simulink model "PI_OL_vs_PI_CC_v2023b"  (R2023b)
settings: Solver=FixedStepDiscrete  StartTime=0.0  StopTime=30  FixedStep=Ts_Power  MaxStep=1e-4  RelTol=1e-3
InitFcn:
  | run PI_VC_vs_PI_CC_ini;
values from neighbouring files (symbols this model uses):
  C = 4e-6    (= 4e-06)    [PI_OL_vs_PI_CC_ini.m]    (also in PI_VC_vs_UPI_CC_ini.m)
  C_2 = 4e-6    (= 4e-06)    [PI_OL_vs_PI_CC_ini.m]    (also in PI_VC_vs_UPI_CC_ini.m)
  K_i_pll = 1.8/0.00251    (= 717.131474104)    [PI_OL_vs_PI_CC_ini.m]    (also in PI_VC_vs_UPI_CC_ini.m)
  K_p_pll = 1.8    [PI_OL_vs_PI_CC_ini.m]    (also in PI_VC_vs_UPI_CC_ini.m)
  L_line_12_13 = X_line_12_13/(2*pi*50)    (= 0.000798957814321)    [PI_OL_vs_PI_CC_ini.m]    (also in PI_VC_vs_UPI_CC_ini.m)
  L_line_13_14 = X_line_13_14/(2*pi*50)    (= 0.000200535228296)    [PI_OL_vs_PI_CC_ini.m]    (also in PI_VC_vs_UPI_CC_ini.m)
  L_s = 1.25e-3    (= 0.00125)    [PI_OL_vs_PI_CC_ini.m]    (also in PI_VC_vs_UPI_CC_ini.m)
  L_s2 = 1.25e-3    (= 0.00125)    [PI_OL_vs_PI_CC_ini.m]    (also in PI_VC_vs_UPI_CC_ini.m)
  L_t = 1.25e-3    (= 0.00125)    [PI_OL_vs_PI_CC_ini.m]    (also in PI_VC_vs_UPI_CC_ini.m)
  L_t2 = 1.25e-3    (= 0.00125)    [PI_OL_vs_PI_CC_ini.m]    (also in PI_VC_vs_UPI_CC_ini.m)
  params_cc = [R_t2;L_t2;R_s2;L_s2;K_pi;Ki_i]    [PI_OL_vs_PI_CC_ini.m]    (also in PI_VC_vs_UPI_CC_ini.m)
  params_pi_cc = [S_b,U_b,K_p,T_p,K_q,T_q,X,R]    [PI_OL_vs_PI_CC_ini.m]    (also in PI_VC_vs_UPI_CC_ini.m)
  params_pi_vc = [S_b,U_b,K_p,T_p,K_q,T_q,Xv,Rv]    [PI_OL_vs_PI_CC_ini.m]    (also in PI_VC_vs_UPI_CC_ini.m)
  R_d = 10    [PI_OL_vs_PI_CC_ini.m]    (also in PI_VC_vs_UPI_CC_ini.m)
  R_d2 = 10    [PI_OL_vs_PI_CC_ini.m]    (also in PI_VC_vs_UPI_CC_ini.m)
  R_line_12_13 = (0.06)*Length    (= 0.24)    [PI_OL_vs_PI_CC_ini.m]    (also in PI_VC_vs_UPI_CC_ini.m)
  R_line_13_14 = (0.025)*Length    (= 0.1)    [PI_OL_vs_PI_CC_ini.m]    (also in PI_VC_vs_UPI_CC_ini.m)
  R_s = L_s*omega/10    (= 0.0392699081699)    [PI_OL_vs_PI_CC_ini.m]    (also in PI_VC_vs_UPI_CC_ini.m)
  R_s2 = L_s*omega/10    (= 0.0392699081699)    [PI_OL_vs_PI_CC_ini.m]    (also in PI_VC_vs_UPI_CC_ini.m)
  R_t = L_t*omega/10    (= 0.0392699081699)    [PI_OL_vs_PI_CC_ini.m]    (also in PI_VC_vs_UPI_CC_ini.m)
  R_t2 = L_t*omega/10    (= 0.0392699081699)    [PI_OL_vs_PI_CC_ini.m]    (also in PI_VC_vs_UPI_CC_ini.m)
  S_b = 20e3    (= 20000)    [PI_OL_vs_PI_CC_ini.m]    (also in PI_VC_vs_UPI_CC_ini.m)
  Ts_Control = 50e-6    (= 5e-05)    [PI_OL_vs_PI_CC_ini.m]    (also in PI_VC_vs_UPI_CC_ini.m)
  Ts_Power = 50e-6    (= 5e-05)    [PI_OL_vs_PI_CC_ini.m]    (also in PI_VC_vs_UPI_CC_ini.m)
  v_dc = 800    [PI_OL_vs_PI_CC_ini.m]    (also in PI_VC_vs_UPI_CC_ini.m)
undefined symbols (not defined in the file or in its folder): DiscIntNeverNeededParam
libraries: spsThreePhaseSeriesRLCBranchLib x10, spsThreePhaseVIMeasurementLib x6, spsFirstOrderFilterLib x4, eeGeneralControl x2, spsPower3phInstantaneousLib x2, spsDCVoltageSourceLib x2, spsUniversalBridgeLib x2, spsVoltageMeasurementLib x2, spsThreePhaseBreakerLib x2, spsRMSLib x1, simulink x1, spsGroundLib x1
settings Model: Creator=Manuel  LastModifiedBy=iberi
settings SolverCC: AlgebraicLoopSolver=TrustRegion
settings DataIOCC: ReturnWorkspaceOutputs=off
settings DebuggingCC: UnconnectedInputMsg=warning  UnconnectedOutputMsg=warning  UnconnectedLineMsg=warning  ArithmeticOperatorsInVariantConditions=warning
settings ModelReferenceCC: EnableRefExpFcnMdlSchedulingChecks=on
settings SFSimCC: SimUseLocalCustomCode=off  CustomCodeUndefinedFunction=UseInterfaceOnly
settings RTWCC: RTWUseLocalCustomCode=off  DLArmComputeVersion=19.05

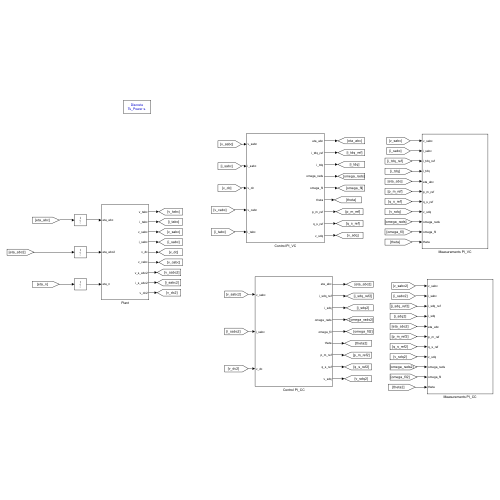
[thumbnail: Simulink's stored preview of the top-level diagram]
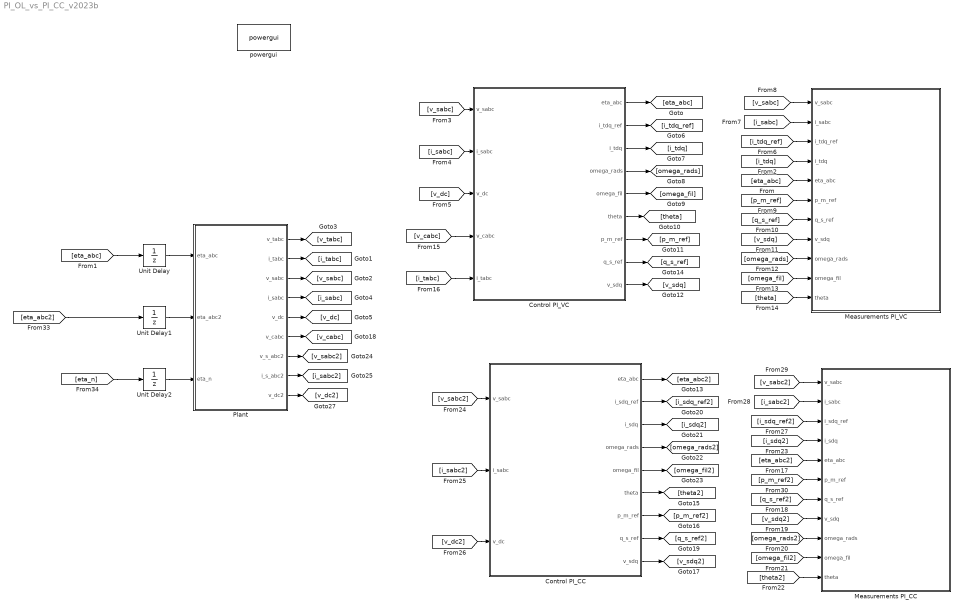
== system PI_OL_vs_PI_CC_v2023b ==
  Control PI_CC : Subsystem
  Control PI_VC : Subsystem
  Measurements PI_CC : Subsystem
  Measurements PI_VC : Subsystem
  Plant : Subsystem
  Unit Delay : UnitDelay  SampleTime=-1  HasFrameUpgradeWarning=on
  Unit Delay1 : UnitDelay  SampleTime=-1  HasFrameUpgradeWarning=on
  Unit Delay2 : UnitDelay  SampleTime=-1  HasFrameUpgradeWarning=on
  powergui : spspowerguiLib/powergui  Priority=1  SimulationMode=Discrete  SampleTime=Ts_Power  frequency=60  Iterations=50  frequencyindice=0  Pbase=100e6  ErrMax=1e-4  UnitsV=kV  UnitsW=MW  buscounter=0  FunctionMessages=off  echomessages=off  EnableUseOfTLC=off  CurrentSourceSwitches=off  DisableSnubberDevices=off  DisableRonSwitches=off  DisableVfSwitches=off  DisplayEquations=off  AutomaticDiscreteSolvers=off  SolverType=Tustin/Backward Euler (TBE)  Interpol=off  ExternalGateDelay=off  methode=off  Ts=100  x0status=blocks  SPID=on  SwTol=0  HookPort=off  NonlinearTolerance=1e-4  nMaxIteration=100  ContinueOnMaxIteration=off  RestoreLinks=warning  ResistiveCurrentMeasurement=off  Frange=[0:2:500]  Ylog=off  Xlog=on  ShowGrid=off  save=off  variable=ZData  structure=v_sabc  ZoomFFT=off  StartTime=4  cycles=5  DisplayStyle=2  fundamental=50  FreqAxis=off  MaxFrequency=10000  frequencyindicesteady=1  RmsSteady=1  display=off
  wires:
  Plant/5(v_dc) -> [v_dc]
  [eta_abc] -> Unit Delay/1
  Plant/1(v_tabc) -> [v_tabc]
  Plant/2(i_tabc) -> [i_tabc]
  Plant/4(i_sabc) -> [i_sabc]
  Plant/3(v_sabc) -> [v_sabc]
  Plant/6(v_cabc) -> [v_cabc]
  [v_sabc] -> Control PI_VC/1(v_sabc)
  [i_sabc] -> Control PI_VC/2(i_sabc)
  [v_dc] -> Control PI_VC/3(v_dc)
  Control PI_VC/1(eta_abc) -> [eta_abc]
  Control PI_VC/2(i_tdq_ref) -> [i_tdq_ref]
  Control PI_VC/3(i_tdq) -> [i_tdq]
  Control PI_VC/4(omega_rads) -> [omega_rads]
  Control PI_VC/5(omega_fil) -> [omega_fil]
  Control PI_VC/6(theta) -> [theta]
  Control PI_VC/7(p_m_ref) -> [p_m_ref]
  Control PI_VC/8(q_s_ref) -> [q_s_ref]
  Control PI_VC/9(v_sdq) -> [v_sdq]
  [eta_abc] -> Measurements PI_VC/5(eta_abc)
  [i_tdq] -> Measurements PI_VC/4(i_tdq)
  [i_tdq_ref] -> Measurements PI_VC/3(i_tdq_ref)
  [i_sabc] -> Measurements PI_VC/2(i_sabc)
  [v_sabc] -> Measurements PI_VC/1(v_sabc)
  [p_m_ref] -> Measurements PI_VC/6(p_m_ref)
  [q_s_ref] -> Measurements PI_VC/7(q_s_ref)
  [v_sdq] -> Measurements PI_VC/8(v_sdq)
  [omega_rads] -> Measurements PI_VC/9(omega_rads)
  [omega_fil] -> Measurements PI_VC/10(omega_fil)
  [theta] -> Measurements PI_VC/11(theta)
  [v_cabc] -> Control PI_VC/4(v_cabc)
  [i_tabc] -> Control PI_VC/5(i_tabc)
  Unit Delay/1 -> Plant/1(eta_abc)
  Unit Delay1/1 -> Plant/2(eta_abc2)
  [eta_n] -> Unit Delay2/1
  Unit Delay2/1 -> Plant/3(eta_n)
  Plant/7(v_s_abc2) -> [v_sabc2]
  Plant/8(i_s_abc2) -> [i_sabc2]
  Plant/9(v_dc2) -> [v_dc2]
  [eta_abc2] -> Unit Delay1/1
  Control PI_CC/9(v_sdq) -> [v_sdq2]
  Control PI_CC/6(theta) -> [theta2]
  Control PI_CC/1(eta_abc) -> [eta_abc2]
  [q_s_ref2] -> Measurements PI_CC/7(q_s_ref)
  Control PI_CC/3(i_sdq) -> [i_sdq2]
  [omega_fil2] -> Measurements PI_CC/10(omega_fil)
  [i_sabc2] -> Control PI_CC/2(i_sabc)
  Control PI_CC/5(omega_fil) -> [omega_fil2]
  [p_m_ref2] -> Measurements PI_CC/6(p_m_ref)
  Control PI_CC/7(p_m_ref) -> [p_m_ref2]
  [i_sdq2] -> Measurements PI_CC/4(i_sdq)
  [v_dc2] -> Control PI_CC/3(v_dc)
  Control PI_CC/4(omega_rads) -> [omega_rads2]
  [eta_abc2] -> Measurements PI_CC/5(eta_abc)
  [v_sdq2] -> Measurements PI_CC/8(v_sdq)
  [theta2] -> Measurements PI_CC/11(theta)
  Control PI_CC/8(q_s_ref) -> [q_s_ref2]
  [v_sabc2] -> Measurements PI_CC/1(v_sabc)
  [omega_rads2] -> Measurements PI_CC/9(omega_rads)
  [i_sabc2] -> Measurements PI_CC/2(i_sabc)
  [i_sdq_ref2] -> Measurements PI_CC/3(i_sdq_ref)
  [v_sabc2] -> Control PI_CC/1(v_sabc)
  Control PI_CC/2(i_sdq_ref) -> [i_sdq_ref2]

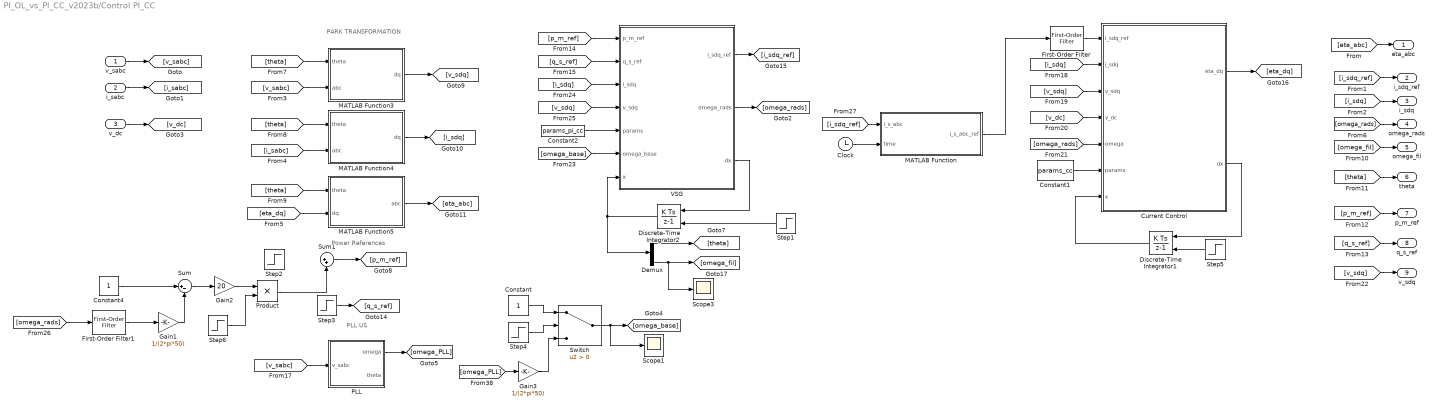
== system PI_OL_vs_PI_CC_v2023b/Control PI_CC ==
  note: PARK TRANSFORMATION
  note: Power References
  note: PLL US
  v_sabc : Inport
  i_sabc : Inport  Port=2
  v_dc : Inport  Port=3
  Clock : Clock
  Constant : Constant
  Constant1 : Constant  Value=params_cc
  Constant2 : Constant  Value=params_pi_cc
  Constant4 : Constant
  Current Control : MATLAB Function  TreatAsAtomicUnit=on
  Demux : Demux
  Discrete-Time Integrator1 : DiscreteIntegrator  ExternalReset=rising  InitialCondition=[0;0]  SampleTime=Ts_Control  ICPrevOutput=DiscIntNeverNeededParam  ICPrevScaledInput=DiscIntNeverNeededParam
  Discrete-Time Integrator2 : DiscreteIntegrator  ExternalReset=rising  InitialCondition=[0;0;0;2*pi*50]  SampleTime=Ts_Control  ICPrevOutput=DiscIntNeverNeededParam  ICPrevScaledInput=DiscIntNeverNeededParam
  First-Order Filter : spsFirstOrderFilterLib/First-Order Filter  FilterType=Lowpass  Tc=2.4e-3  Ts=Ts_Control  Initialize=on  Vac_Init=[0, 0, 60]  Vdc_Init=0  PlotResponse=off  FreqRange="[0,  200,  1]"
  First-Order Filter1 : spsFirstOrderFilterLib/First-Order Filter  FilterType=Lowpass  Tc=10e-3  Ts=Ts_Control  Initialize=on  Vac_Init=[0, 0, 60]  Vdc_Init=0  PlotResponse=off  FreqRange="[0,  200,  1]"
  Gain1 : Gain  Gain=1/(2*pi*50)
  Gain2 : Gain  Gain=20
  Gain3 : Gain  Gain=1/(2*pi*50)
  MATLAB Function : MATLAB Function  TreatAsAtomicUnit=on
  MATLAB Function3 : MATLAB Function  TreatAsAtomicUnit=on
  MATLAB Function4 : MATLAB Function  TreatAsAtomicUnit=on
  MATLAB Function5 : MATLAB Function  TreatAsAtomicUnit=on
  PLL : Subsystem
  Product : Product
  Scope1 : Scope
  Scope3 : Scope
  Step1 : Step  SampleTime=0
  Step2 : Step  Time=4  After=0.1  SampleTime=0
  Step3 : Step  Time=12  After=0  SampleTime=0
  Step4 : Step  Time=2  SampleTime=0
  Step5 : Step  SampleTime=0
  Step6 : Step  SampleTime=0
  Sum : Sum  Inputs=|+-
  Sum1 : Sum  Inputs=|++
  Switch : Switch  Criteria=u2 > Threshold  SaturateOnIntegerOverflow=off  InputSameDT=off
  VSG : MATLAB Function  TreatAsAtomicUnit=on
  eta_abc : Outport  VectorParamsAs1DForOutWhenUnconnected=off
  i_sdq_ref : Outport  Port=2  VectorParamsAs1DForOutWhenUnconnected=off
  i_sdq : Outport  Port=3  VectorParamsAs1DForOutWhenUnconnected=off
  omega_rads : Outport  Port=4  VectorParamsAs1DForOutWhenUnconnected=off
  omega_fil : Outport  Port=5  VectorParamsAs1DForOutWhenUnconnected=off
  theta : Outport  Port=6  VectorParamsAs1DForOutWhenUnconnected=off
  p_m_ref : Outport  Port=7  VectorParamsAs1DForOutWhenUnconnected=off
  q_s_ref : Outport  Port=8  VectorParamsAs1DForOutWhenUnconnected=off
  v_sdq : Outport  Port=9  VectorParamsAs1DForOutWhenUnconnected=off
  wires:
  [theta] -> MATLAB Function4/1(theta)
  MATLAB Function5/1(abc) -> [eta_abc]
  [i_sabc] -> MATLAB Function4/2(abc)
  [eta_dq] -> MATLAB Function5/2(dq)
  MATLAB Function3/1(dq) -> [v_sdq]
  MATLAB Function4/1(dq) -> [i_sdq]
  [theta] -> MATLAB Function5/1(theta)
  [theta] -> MATLAB Function3/1(theta)
  Step3/1 -> [q_s_ref]
  [v_sabc] -> MATLAB Function3/2(abc)
  Discrete-Time Integrator2/1 -> Demux/1, VSG/7(x)
  [i_sdq] -> VSG/3(i_sdq)
  Demux/4 -> Scope3/1, [omega_fil]
  Demux/1 -> [theta]
  [v_dc] -> Current Control/4(v_dc)
  [v_sdq] -> VSG/4(v_sdq)
  Constant2/1 -> VSG/5(params)
  [p_m_ref] -> VSG/1(p_m_ref)
  Constant1/1 -> Current Control/6(params)
  Current Control/1(eta_dq) -> [eta_dq]
  MATLAB Function/1(i_s_abc_ref) -> First-Order Filter/1
  [omega_rads] -> Current Control/5(omega)
  Current Control/2(dx) -> Discrete-Time Integrator1/1
  [q_s_ref] -> VSG/2(q_s_ref)
  Discrete-Time Integrator1/1 -> Current Control/7(x)
  VSG/3(dx) -> Discrete-Time Integrator2/1
  VSG/1(i_sdq_ref) -> [i_sdq_ref]
  [v_sdq] -> Current Control/3(v_sdq)
  [i_sdq] -> Current Control/2(i_sdq)
  v_sabc/1 -> [v_sabc]
  i_sabc/1 -> [i_sabc]
  VSG/2(omega_rads) -> [omega_rads]
  v_dc/1 -> [v_dc]
  [eta_abc] -> eta_abc/1
  [i_sdq_ref] -> i_sdq_ref/1
  [i_sdq] -> i_sdq/1
  [omega_rads] -> omega_rads/1
  [omega_fil] -> omega_fil/1
  [theta] -> theta/1
  [p_m_ref] -> p_m_ref/1
  [q_s_ref] -> q_s_ref/1
  [v_sabc] -> PLL/1(v_sabc)
  [v_sdq] -> v_sdq/1
  Switch/1 -> Scope1/1, [omega_base]
  Constant/1 -> Switch/1
  Gain3/1 -> Switch/3
  [omega_PLL] -> Gain3/1
  Step4/1 -> Switch/2
  PLL/1(omega) -> [omega_PLL]
  [omega_base] -> VSG/6(omega_base)
  First-Order Filter/1 -> Current Control/1(i_sdq_ref)
  Step1/1 -> Discrete-Time Integrator2/2
  Step5/1 -> Discrete-Time Integrator1/2
  Gain1/1 -> Sum/2
  Constant4/1 -> Sum/1
  Sum/1 -> Gain2/1
  [omega_rads] -> First-Order Filter1/1
  Sum1/1 -> [p_m_ref]
  Gain2/1 -> Product/1
  Step6/1 -> Product/2
  Product/1 -> Sum1/2
  Clock/1 -> MATLAB Function/2(time)
  [i_sdq_ref] -> MATLAB Function/1(i_s_abc)
  First-Order Filter1/1 -> Gain1/1

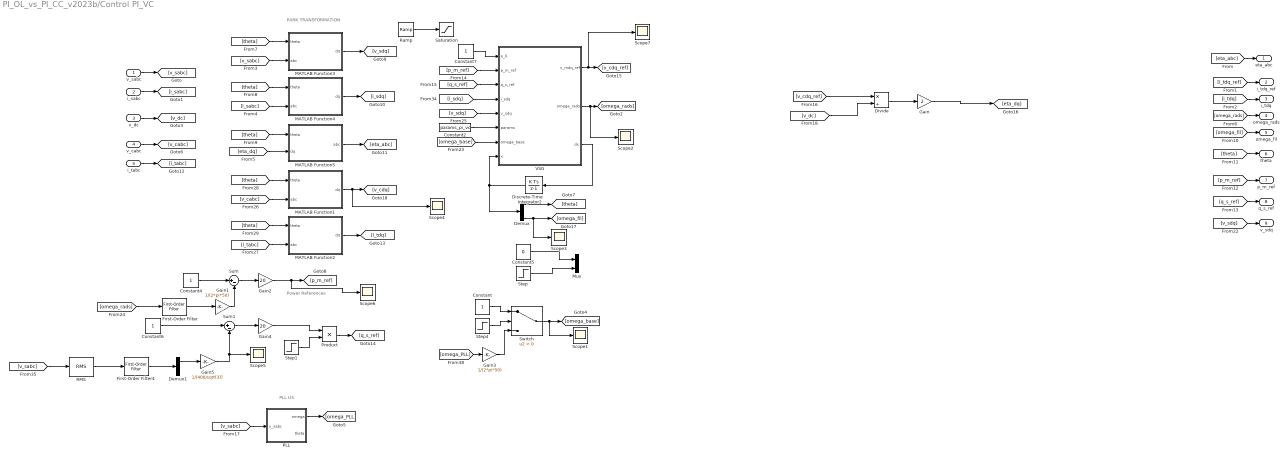
== system PI_OL_vs_PI_CC_v2023b/Control PI_VC ==
  note: PARK TRANSFORMATION
  note: Power References
  note: PLL US
  v_sabc : Inport
  i_sabc : Inport  Port=2
  v_dc : Inport  Port=3
  v_cabc : Inport  Port=4
  i_tabc : Inport  Port=5
  Constant{,4,6..7} (4 alike) : Constant
  Constant2 : Constant  Value=params_pi_vc
  Constant5 : Constant  Value=0
  Demux : Demux
  Demux1 : Demux  Outputs=3
  Discrete-Time Integrator2 : DiscreteIntegrator  InitialCondition=[0;0;0;2*pi*50]  SampleTime=Ts_Control  ICPrevOutput=DiscIntNeverNeededParam  ICPrevScaledInput=DiscIntNeverNeededParam
  Divide : Product  Inputs=*/
  First-Order Filter : spsFirstOrderFilterLib/First-Order Filter  FilterType=Lowpass  Tc=10e-3  Ts=Ts_Control  Initialize=on  Vac_Init=[0, 0, 60]  Vdc_Init=0  PlotResponse=off  FreqRange="[0,  200,  1]"
  First-Order Filter4 : spsFirstOrderFilterLib/First-Order Filter  FilterType=Lowpass  Tc=10e-3  Ts=Ts_Control  Initialize=on  Vac_Init=[0, 0, 60]  Vdc_Init=0  PlotResponse=off  FreqRange="[0,  200,  1]"
  Gain : Gain  Gain=2
  Gain1 : Gain  Gain=1/(2*pi*50)
  Gain2 : Gain  Gain=20
  Gain3 : Gain  Gain=1/(2*pi*50)
  Gain4 : Gain  Gain=20
  Gain5 : Gain  Gain=1/(400/sqrt(3))
  MATLAB Function1 : MATLAB Function  TreatAsAtomicUnit=on
  MATLAB Function2 : MATLAB Function  TreatAsAtomicUnit=on
  MATLAB Function3 : MATLAB Function  TreatAsAtomicUnit=on
  MATLAB Function4 : MATLAB Function  TreatAsAtomicUnit=on
  MATLAB Function5 : MATLAB Function  TreatAsAtomicUnit=on
  Mux : Mux  Inputs=2
  PLL : Subsystem
  Product : Product
  RMS : spsRMSLib/RMS  TrueRMS=on  Freq=50  RMSInit=230  Ts=Ts_Control
  Ramp : simulink/Sources/Ramp  slope=1  start=0  InitialOutput=0
  Saturation : Saturate  UpperLimit=1  LowerLimit=-1
  Scope{1..7} (7 alike) : Scope
  Step : Step  After=-325  SampleTime=0
  Step1 : Step  Time=0  SampleTime=0
  Step4 : Step  Time=0  SampleTime=0
  Sum : Sum  Inputs=|+-
  Sum1 : Sum  Inputs=|+-
  Switch : Switch  Criteria=u2 > Threshold  SaturateOnIntegerOverflow=off  InputSameDT=off
  VSG : MATLAB Function  TreatAsAtomicUnit=on
  eta_abc : Outport  VectorParamsAs1DForOutWhenUnconnected=off
  i_tdq_ref : Outport  Port=2  VectorParamsAs1DForOutWhenUnconnected=off
  i_tdq : Outport  Port=3  VectorParamsAs1DForOutWhenUnconnected=off
  omega_rads : Outport  Port=4  VectorParamsAs1DForOutWhenUnconnected=off
  omega_fil : Outport  Port=5  VectorParamsAs1DForOutWhenUnconnected=off
  theta : Outport  Port=6  VectorParamsAs1DForOutWhenUnconnected=off
  p_m_ref : Outport  Port=7  VectorParamsAs1DForOutWhenUnconnected=off
  q_s_ref : Outport  Port=8  VectorParamsAs1DForOutWhenUnconnected=off
  v_sdq : Outport  Port=9  VectorParamsAs1DForOutWhenUnconnected=off
  wires:
  [theta] -> MATLAB Function4/1(theta)
  MATLAB Function5/1(abc) -> [eta_abc]
  [i_sabc] -> MATLAB Function4/2(abc)
  [eta_dq] -> MATLAB Function5/2(dq)
  Gain2/1 -> Scope6/1, [p_m_ref]
  MATLAB Function3/1(dq) -> [v_sdq]
  MATLAB Function4/1(dq) -> [i_sdq]
  [theta] -> MATLAB Function5/1(theta)
  [theta] -> MATLAB Function3/1(theta)
  [v_sabc] -> MATLAB Function3/2(abc)
  Discrete-Time Integrator2/1 -> Demux/1, VSG/8(x)
  Demux/4 -> Scope3/1, [omega_fil]
  Demux/1 -> [theta]
  Constant2/1 -> VSG/6(params)
  [p_m_ref] -> VSG/2(p_m_ref)
  Gain/1 -> [eta_dq]
  [q_s_ref] -> VSG/3(q_s_ref)
  VSG/3(dx) -> Discrete-Time Integrator2/1
  v_sabc/1 -> [v_sabc]
  i_sabc/1 -> [i_sabc]
  VSG/2(omega_rads) -> Scope2/1, [omega_rads]
  v_dc/1 -> [v_dc]
  [eta_abc] -> eta_abc/1
  [i_tdq_ref] -> i_tdq_ref/1
  [i_tdq] -> i_tdq/1
  [omega_rads] -> omega_rads/1
  [omega_fil] -> omega_fil/1
  [theta] -> theta/1
  [p_m_ref] -> p_m_ref/1
  [q_s_ref] -> q_s_ref/1
  [v_sabc] -> PLL/1(v_sabc)
  [v_sdq] -> v_sdq/1
  Switch/1 -> Scope1/1, [omega_base]
  Constant/1 -> Switch/1
  Gain3/1 -> Switch/3
  [omega_PLL] -> Gain3/1
  Step4/1 -> Switch/2
  PLL/1(omega) -> [omega_PLL]
  [omega_base] -> VSG/7(omega_base)
  i_tabc/1 -> [i_tabc]
  v_cabc/1 -> [v_cabc]
  [v_cabc] -> MATLAB Function1/2(abc)
  [theta] -> MATLAB Function1/1(theta)
  MATLAB Function2/1(dq) -> [i_tdq]
  MATLAB Function1/1(dq) -> Scope4/1, [v_cdq]
  [i_tabc] -> MATLAB Function2/2(abc)
  [theta] -> MATLAB Function2/1(theta)
  [i_sdq] -> VSG/4(i_sdq)
  [v_sdq] -> VSG/5(v_sdq)
  Constant5/1 -> Mux/1
  Step/1 -> Mux/2
  [omega_rads] -> First-Order Filter/1
  Gain1/1 -> Sum/2
  Sum/1 -> Gain2/1
  Sum1/1 -> Gain4/1
  VSG/1(v_mdq_ref) -> Scope7/1, [v_cdq_ref]
  [v_sabc] -> RMS/1
  RMS/1 -> First-Order Filter4/1
  Demux1/1 -> Gain5/1
  Gain5/1 -> Scope5/1, Sum1/2
  Constant4/1 -> Sum/1
  Ramp/1 -> Saturation/1
  Constant6/1 -> Sum1/1
  Product/1 -> [q_s_ref]
  Gain4/1 -> Product/1
  Step1/1 -> Product/2
  Constant7/1 -> VSG/1(e_0)
  First-Order Filter/1 -> Gain1/1
  First-Order Filter4/1 -> Demux1/1
  [v_cdq_ref] -> Divide/1
  [v_dc] -> Divide/2
  Divide/1 -> Gain/1

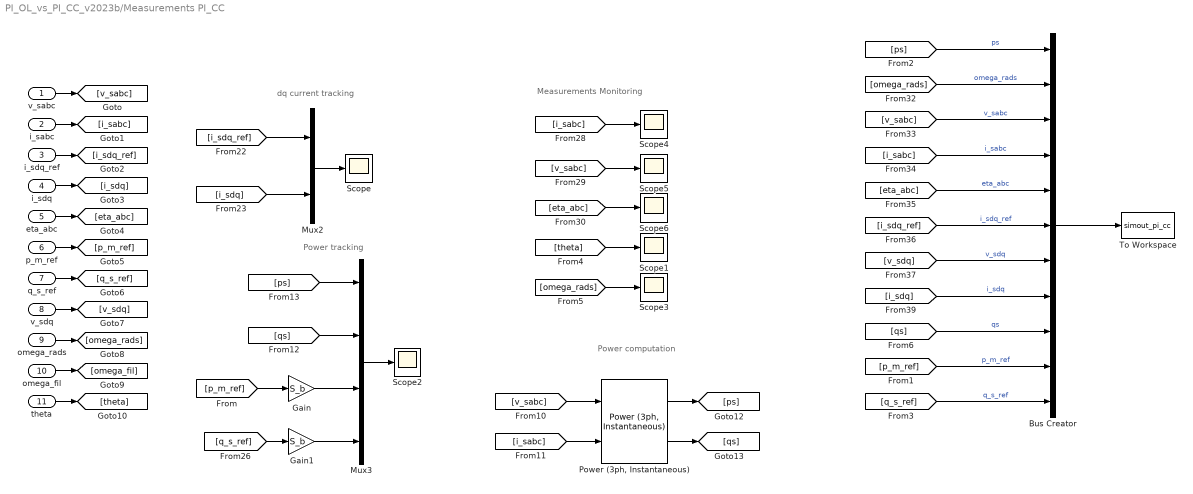
== system PI_OL_vs_PI_CC_v2023b/Measurements PI_CC ==
  note: Power computation
  note: dq current tracking
  note: Measurements Monitoring
  note: Power tracking
  v_sabc : Inport
  i_sabc : Inport  Port=2
  i_sdq_ref : Inport  Port=3
  i_sdq : Inport  Port=4
  eta_abc : Inport  Port=5
  p_m_ref : Inport  Port=6
  q_s_ref : Inport  Port=7
  v_sdq : Inport  Port=8
  omega_rads : Inport  Port=9
  omega_fil : Inport  Port=10
  theta : Inport  Port=11
  Bus Creator : BusCreator  Inputs=11
  Gain : Gain  Gain=S_b
  Gain1 : Gain  Gain=S_b
  Mux2 : Mux  Inputs=2
  Mux3 : Mux
  "Power (3ph, Instantaneous)" : spsPower3phInstantaneousLib/Power (3ph, Instantaneous)
  Scope{,1..6} (7 alike) : Scope
  To Workspace : ToWorkspace  VariableName=simout_pi_cc  SaveFormat=Timeseries  SampleTime=-1
  wires:
  [v_sdq] -> Bus Creator/7  "v_sdq"
  [i_sdq] -> Mux2/2
  [v_sabc] -> "Power (3ph, Instantaneous)"/1
  Mux2/1 -> Scope/1
  Gain1/1 -> Mux3/4
  Bus Creator/1 -> To Workspace/1
  [qs] -> Mux3/2
  [eta_abc] -> Scope6/1
  [omega_rads] -> Bus Creator/2  "omega_rads"
  [i_sdq] -> Bus Creator/8  "i_sdq"
  [i_sdq_ref] -> Mux2/1
  [p_m_ref] -> Gain/1
  [v_sabc] -> Bus Creator/3  "v_sabc"
  [ps] -> Bus Creator/1  "ps"
  [v_sabc] -> Scope5/1
  [i_sabc] -> "Power (3ph, Instantaneous)"/2
  "Power (3ph, Instantaneous)"/1 -> [ps]
  [i_sabc] -> Scope4/1
  "Power (3ph, Instantaneous)"/2 -> [qs]
  [q_s_ref] -> Gain1/1
  [eta_abc] -> Bus Creator/5  "eta_abc"
  [ps] -> Mux3/1
  [qs] -> Bus Creator/9  "qs"
  Gain/1 -> Mux3/3
  [i_sabc] -> Bus Creator/4  "i_sabc"
  Mux3/1 -> Scope2/1
  [i_sdq_ref] -> Bus Creator/6  "i_sdq_ref"
  v_sabc/1 -> [v_sabc]
  i_sabc/1 -> [i_sabc]
  i_sdq_ref/1 -> [i_sdq_ref]
  i_sdq/1 -> [i_sdq]
  eta_abc/1 -> [eta_abc]
  p_m_ref/1 -> [p_m_ref]
  q_s_ref/1 -> [q_s_ref]
  v_sdq/1 -> [v_sdq]
  omega_rads/1 -> [omega_rads]
  omega_fil/1 -> [omega_fil]
  [p_m_ref] -> Bus Creator/10  "p_m_ref"
  [q_s_ref] -> Bus Creator/11  "q_s_ref"
  theta/1 -> [theta]
  [theta] -> Scope1/1
  [omega_rads] -> Scope3/1

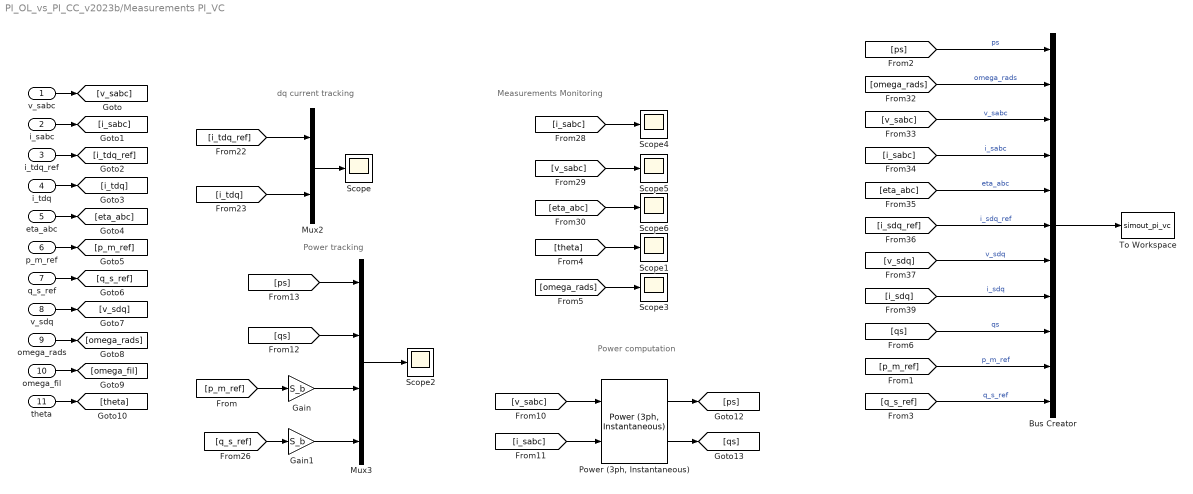
== system PI_OL_vs_PI_CC_v2023b/Measurements PI_VC ==
  note: Power computation
  note: dq current tracking
  note: Measurements Monitoring
  note: Power tracking
  v_sabc : Inport
  i_sabc : Inport  Port=2
  i_tdq_ref : Inport  Port=3
  i_tdq : Inport  Port=4
  eta_abc : Inport  Port=5
  p_m_ref : Inport  Port=6
  q_s_ref : Inport  Port=7
  v_sdq : Inport  Port=8
  omega_rads : Inport  Port=9
  omega_fil : Inport  Port=10
  theta : Inport  Port=11
  Bus Creator : BusCreator  Inputs=11
  Gain : Gain  Gain=S_b
  Gain1 : Gain  Gain=S_b
  Mux2 : Mux  Inputs=2
  Mux3 : Mux
  "Power (3ph, Instantaneous)" : spsPower3phInstantaneousLib/Power (3ph, Instantaneous)
  Scope{,1..6} (7 alike) : Scope
  To Workspace : ToWorkspace  VariableName=simout_pi_vc  SaveFormat=Timeseries  SampleTime=-1
  wires:
  [v_sdq] -> Bus Creator/7  "v_sdq"
  [i_tdq] -> Mux2/2
  [v_sabc] -> "Power (3ph, Instantaneous)"/1
  Mux2/1 -> Scope/1
  Gain1/1 -> Mux3/4
  Bus Creator/1 -> To Workspace/1
  [qs] -> Mux3/2
  [eta_abc] -> Scope6/1
  [omega_rads] -> Bus Creator/2  "omega_rads"
  [i_sdq] -> Bus Creator/8  "i_sdq"
  [i_tdq_ref] -> Mux2/1
  [p_m_ref] -> Gain/1
  [v_sabc] -> Bus Creator/3  "v_sabc"
  [ps] -> Bus Creator/1  "ps"
  [v_sabc] -> Scope5/1
  [i_sabc] -> "Power (3ph, Instantaneous)"/2
  "Power (3ph, Instantaneous)"/1 -> [ps]
  [i_sabc] -> Scope4/1
  "Power (3ph, Instantaneous)"/2 -> [qs]
  [q_s_ref] -> Gain1/1
  [eta_abc] -> Bus Creator/5  "eta_abc"
  [ps] -> Mux3/1
  [qs] -> Bus Creator/9  "qs"
  Gain/1 -> Mux3/3
  [i_sabc] -> Bus Creator/4  "i_sabc"
  Mux3/1 -> Scope2/1
  [i_sdq_ref] -> Bus Creator/6  "i_sdq_ref"
  v_sabc/1 -> [v_sabc]
  i_sabc/1 -> [i_sabc]
  i_tdq_ref/1 -> [i_tdq_ref]
  i_tdq/1 -> [i_tdq]
  eta_abc/1 -> [eta_abc]
  p_m_ref/1 -> [p_m_ref]
  q_s_ref/1 -> [q_s_ref]
  v_sdq/1 -> [v_sdq]
  omega_rads/1 -> [omega_rads]
  omega_fil/1 -> [omega_fil]
  [p_m_ref] -> Bus Creator/10  "p_m_ref"
  [q_s_ref] -> Bus Creator/11  "q_s_ref"
  theta/1 -> [theta]
  [theta] -> Scope1/1
  [omega_rads] -> Scope3/1

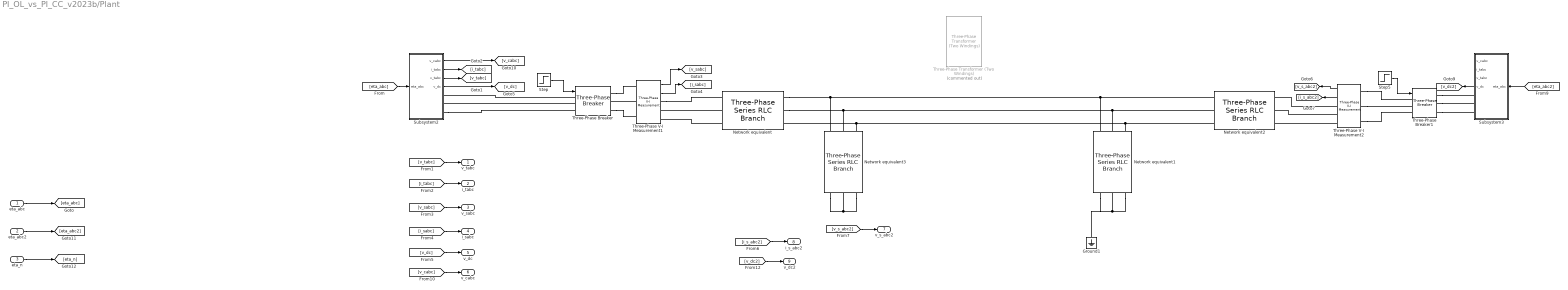
== system PI_OL_vs_PI_CC_v2023b/Plant ==
  eta_abc : Inport
  eta_abc2 : Inport  Port=2
  eta_n : Inport  Port=3
  Ground1 : spsGroundLib/Ground  LConnTagsString=a
  Network equivalent : spsThreePhaseSeriesRLCBranchLib/Three-Phase Series RLC Branch  LConnTagsString=A|B|C  RConnTagsString=A|B|C  BranchType=RL  Resistance=R_line_12_13  Inductance=L_line_12_13  Capacitance=1e-6  Measurements=None
  Network equivalent1 : spsThreePhaseSeriesRLCBranchLib/Three-Phase Series RLC Branch  LConnTagsString=A|B|C  RConnTagsString=A|B|C  BranchType=R  Resistance=50  Inductance=L_line_13_14  Capacitance=1e-6  Measurements=None
  Network equivalent2 : spsThreePhaseSeriesRLCBranchLib/Three-Phase Series RLC Branch  LConnTagsString=A|B|C  RConnTagsString=A|B|C  BranchType=RL  Resistance=R_line_13_14  Inductance=L_line_13_14  Capacitance=1e-6  Measurements=None
  Network equivalent3 : spsThreePhaseSeriesRLCBranchLib/Three-Phase Series RLC Branch  LConnTagsString=A|B|C  RConnTagsString=A|B|C  BranchType=R  Resistance=50  Inductance=L_line_13_14  Capacitance=1e-6  Measurements=None
  Step : Step  Time=0  SampleTime=0
  Step5 : Step  SampleTime=0
  Subsystem2 : Subsystem
  Subsystem3 : Subsystem
  Three-Phase Transformer (Two Windings) : spsThreePhaseTransformerTwoWindingsLib/Three-Phase Transformer (Two Windings)  Commented=on  Winding1Connection=Yn  Winding2Connection=Yn  CoreType=Three single-phase transformers  SetSaturation=off  Hysteresis=off  DataFile='hysteresis'  SetInitialFlux=off  Measurements=None  UNITS=pu  NominalPower=[ 125e3 , 50 ]  Winding1=[ 400 , 0.002 , 0.08 ]  Winding2=[ 400 , 0.002 , 0.08 ]  Rm=500  Lm=500  L0=0.5  Saturation=[ 0,0 ; 0.0024,1.2 ; 1.0,1.52 ]  InitialFluxes=[ 0.8 , -0.8 , 0.7 ]  BreakLoop=off  DiscreteSolver=Trapezoidal iterative  DataType=off  TransfoNumber=1
  Three-Phase V-I Measurement1 : spsThreePhaseVIMeasurementLib/Three-Phase V-I Measurement  VoltageMeasurement=phase-to-ground  SetLabelV=off  LabelV=Vabc  Vpu=off  VpuLL=off  CurrentMeasurement=yes  SetLabelI=off  LabelI=Iabc  Ipu=off  Pbase=100e6  Vbase=500e3  OutputType=Complex  PhasorSimulation=off  PSBequivalent=0
  Three-Phase V-I Measurement2 : spsThreePhaseVIMeasurementLib/Three-Phase V-I Measurement  VoltageMeasurement=phase-to-ground  SetLabelV=off  LabelV=Vabc  Vpu=off  VpuLL=off  CurrentMeasurement=yes  SetLabelI=off  LabelI=Iabc  Ipu=off  Pbase=100e6  Vbase=500e3  OutputType=Complex  PhasorSimulation=off  PSBequivalent=0
  Three-Phase Breaker : spsThreePhaseBreakerLib/Three-Phase Breaker  InitialState=open  SwitchA=on  SwitchB=on  SwitchC=on  SwitchTimes="[1/60  5/60]"  External=on  BreakerResistance=0.01  SnubberResistance=1e6  SnubberCapacitance=inf  Measurements=None
  Three-Phase Breaker1 : spsThreePhaseBreakerLib/Three-Phase Breaker  InitialState=open  SwitchA=on  SwitchB=on  SwitchC=on  SwitchTimes="[1/60  5/60]"  External=on  BreakerResistance=0.01  SnubberResistance=1e6  SnubberCapacitance=inf  Measurements=None
  v_tabc : Outport  VectorParamsAs1DForOutWhenUnconnected=off
  i_tabc : Outport  Port=2  VectorParamsAs1DForOutWhenUnconnected=off
  v_sabc : Outport  Port=3  VectorParamsAs1DForOutWhenUnconnected=off
  i_sabc : Outport  Port=4  VectorParamsAs1DForOutWhenUnconnected=off
  v_dc : Outport  Port=5  VectorParamsAs1DForOutWhenUnconnected=off
  v_cabc : Outport  Port=6  VectorParamsAs1DForOutWhenUnconnected=off
  v_s_abc2 : Outport  Port=7  VectorParamsAs1DForOutWhenUnconnected=off
  i_s_abc2 : Outport  Port=8  VectorParamsAs1DForOutWhenUnconnected=off
  v_dc2 : Outport  Port=9  VectorParamsAs1DForOutWhenUnconnected=off
  wires:
  Three-Phase V-I Measurement1/1 -> [v_sabc]
  Three-Phase V-I Measurement1/2 -> [i_sabc]
  [v_tabc] -> v_tabc/1
  [i_tabc] -> i_tabc/1
  [v_sabc] -> v_sabc/1
  [i_sabc] -> i_sabc/1
  eta_abc/1 -> [eta_abc]
  [v_dc] -> v_dc/1
  [v_cabc] -> v_cabc/1
  Step/1 -> Three-Phase Breaker/1
  Three-Phase V-I Measurement2/2 -> [i_s_abc2]
  Three-Phase V-I Measurement2/1 -> [v_s_abc2]
  Step5/1 -> Three-Phase Breaker1/1
  [i_s_abc2] -> i_s_abc2/1
  [v_s_abc2] -> v_s_abc2/1
  eta_abc2/1 -> [eta_abc2]
  eta_n/1 -> [eta_n]
  [v_dc2] -> v_dc2/1
  [eta_abc] -> Subsystem2/1(eta_abc)
  Subsystem2/1(v_cabc) -> [v_cabc]
  Subsystem2/2(i_tabc) -> [i_tabc]
  Subsystem2/3(v_tabc) -> [v_tabc]
  Subsystem2/4(v_dc) -> [v_dc]
  [eta_abc2] -> Subsystem3/1(eta_abc)
  Subsystem3/4(v_dc) -> [v_dc2]
  connections:
  Three-Phase Breaker/RConn3 -- Three-Phase V-I Measurement1/LConn3
  Three-Phase V-I Measurement1/LConn2 -- Three-Phase Breaker/RConn2
  Three-Phase Breaker/RConn1 -- Three-Phase V-I Measurement1/LConn1
  Network equivalent1/RConn3 -- Ground1/LConn1 -- Network equivalent1/RConn1 -- Network equivalent1/RConn2
  Three-Phase Breaker1/RConn2 -- Subsystem3/RConn2
  Three-Phase Breaker1/RConn3 -- Subsystem3/RConn3
  Three-Phase Breaker1/RConn1 -- Subsystem3/RConn1
  Three-Phase V-I Measurement2/LConn2 -- Three-Phase Breaker1/LConn2
  Three-Phase V-I Measurement2/LConn3 -- Three-Phase Breaker1/LConn3
  Three-Phase V-I Measurement2/LConn1 -- Three-Phase Breaker1/LConn1
  Three-Phase V-I Measurement2/RConn2 -- Network equivalent2/RConn2
  Three-Phase V-I Measurement2/RConn3 -- Network equivalent2/RConn3
  Three-Phase V-I Measurement2/RConn1 -- Network equivalent2/RConn1
  Three-Phase Breaker/LConn1 -- Subsystem2/RConn1
  Three-Phase Breaker/LConn2 -- Subsystem2/RConn2
  Subsystem2/RConn3 -- Three-Phase Breaker/LConn3
  Network equivalent/LConn2 -- Three-Phase V-I Measurement1/RConn2
  Network equivalent/LConn3 -- Three-Phase V-I Measurement1/RConn3
  Three-Phase V-I Measurement1/RConn1 -- Network equivalent/LConn1
  Network equivalent1/LConn2 -- Network equivalent3/LConn2 -- Network equivalent/RConn2 -- Network equivalent2/LConn2
  Network equivalent1/LConn3 -- Network equivalent3/LConn3 -- Network equivalent/RConn3 -- Network equivalent2/LConn3
  Network equivalent1/LConn1 -- Network equivalent3/LConn1 -- Network equivalent/RConn1 -- Network equivalent2/LConn1
  Network equivalent3/RConn3 -- Network equivalent3/RConn2 -- Network equivalent3/RConn1

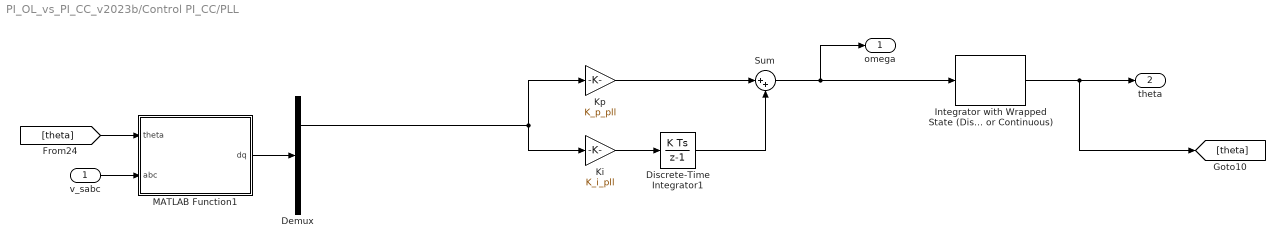
== system PI_OL_vs_PI_CC_v2023b/Control PI_CC/PLL ==
  v_sabc : Inport
  Demux : Demux  Outputs=2
  Discrete-Time Integrator1 : DiscreteIntegrator  SampleTime=Ts_Control  ICPrevOutput=DiscIntNeverNeededParam  ICPrevScaledInput=DiscIntNeverNeededParam
  Integrator with Wrapped State (Discrete or Continuous) : eeGeneralControl/Integrator with Wrapped State (Discrete or Continuous)  LabelModeActiveChoice=Discrete  WrappedStateUpperValue=2*pi  WrappedStateLowerValue=0  x0=0  Ts=Ts_Control
  Ki : Gain  Gain=K_i_pll
  Kp : Gain  Gain=K_p_pll
  MATLAB Function1 : MATLAB Function  TreatAsAtomicUnit=on
  Sum : Sum  Inputs=|++
  omega : Outport  VectorParamsAs1DForOutWhenUnconnected=off
  theta : Outport  Port=2  VectorParamsAs1DForOutWhenUnconnected=off
  wires:
  MATLAB Function1/1(dq) -> Demux/1
  v_sabc/1 -> MATLAB Function1/2(abc)
  [theta] -> MATLAB Function1/1(theta)
  Ki/1 -> Discrete-Time Integrator1/1
  Kp/1 -> Sum/1
  Discrete-Time Integrator1/1 -> Sum/2
  Sum/1 -> Integrator with Wrapped State (Discrete or Continuous)/1, omega/1
  Integrator with Wrapped State (Discrete or Continuous)/1 -> [theta], theta/1
  Demux/1 -> Ki/1, Kp/1

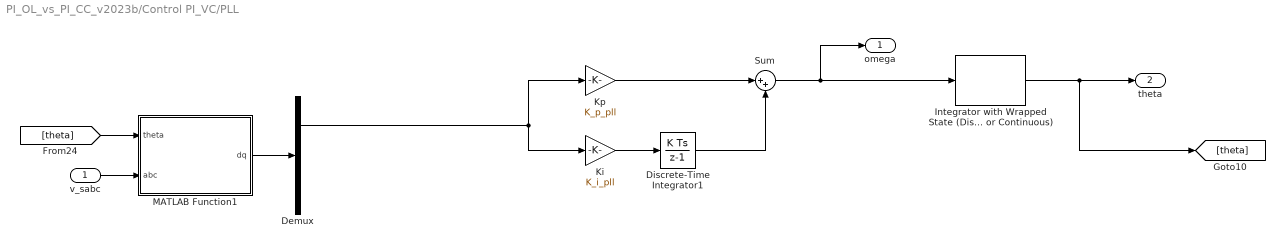
== system PI_OL_vs_PI_CC_v2023b/Control PI_VC/PLL ==
  v_sabc : Inport
  Demux : Demux  Outputs=2
  Discrete-Time Integrator1 : DiscreteIntegrator  SampleTime=Ts_Control  ICPrevOutput=DiscIntNeverNeededParam  ICPrevScaledInput=DiscIntNeverNeededParam
  Integrator with Wrapped State (Discrete or Continuous) : eeGeneralControl/Integrator with Wrapped State (Discrete or Continuous)  LabelModeActiveChoice=Discrete  WrappedStateUpperValue=2*pi  WrappedStateLowerValue=0  x0=0  Ts=Ts_Control
  Ki : Gain  Gain=K_i_pll
  Kp : Gain  Gain=K_p_pll
  MATLAB Function1 : MATLAB Function  TreatAsAtomicUnit=on
  Sum : Sum  Inputs=|++
  omega : Outport  VectorParamsAs1DForOutWhenUnconnected=off
  theta : Outport  Port=2  VectorParamsAs1DForOutWhenUnconnected=off
  wires:
  MATLAB Function1/1(dq) -> Demux/1
  v_sabc/1 -> MATLAB Function1/2(abc)
  [theta] -> MATLAB Function1/1(theta)
  Ki/1 -> Discrete-Time Integrator1/1
  Kp/1 -> Sum/1
  Discrete-Time Integrator1/1 -> Sum/2
  Sum/1 -> Integrator with Wrapped State (Discrete or Continuous)/1, omega/1
  Integrator with Wrapped State (Discrete or Continuous)/1 -> [theta], theta/1
  Demux/1 -> Ki/1, Kp/1

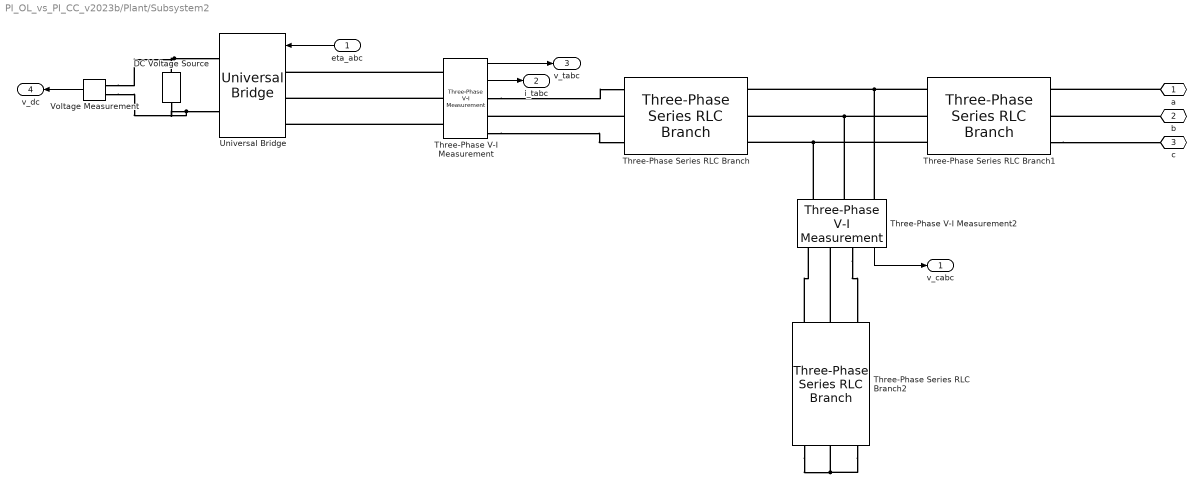
== system PI_OL_vs_PI_CC_v2023b/Plant/Subsystem2 ==
  eta_abc : Inport
  DC Voltage Source : spsDCVoltageSourceLib/DC Voltage Source  Amplitude=v_dc  Measurements=None
  Three-Phase Series RLC Branch : spsThreePhaseSeriesRLCBranchLib/Three-Phase Series RLC Branch  LConnTagsString=A|B|C  RConnTagsString=A|B|C  BranchType=RL  Resistance=R_t  Inductance=L_t  Capacitance=1e-6  Measurements=None
  Three-Phase Series RLC Branch1 : spsThreePhaseSeriesRLCBranchLib/Three-Phase Series RLC Branch  LConnTagsString=A|B|C  RConnTagsString=A|B|C  BranchType=RL  Resistance=R_s  Inductance=L_s  Capacitance=1e-6  Measurements=None
  Three-Phase Series RLC Branch2 : spsThreePhaseSeriesRLCBranchLib/Three-Phase Series RLC Branch  LConnTagsString=A|B|C  RConnTagsString=A|B|C  BranchType=RC  Resistance=R_d  Inductance=L_t  Capacitance=C  Measurements=None
  Three-Phase V-I Measurement : spsThreePhaseVIMeasurementLib/Three-Phase V-I Measurement  VoltageMeasurement=phase-to-ground  SetLabelV=off  LabelV=Vabc  Vpu=off  VpuLL=off  CurrentMeasurement=yes  SetLabelI=off  LabelI=Iabc  Ipu=off  Pbase=100e6  Vbase=500e3  OutputType=Complex  PhasorSimulation=off  PSBequivalent=0
  Three-Phase V-I Measurement2 : spsThreePhaseVIMeasurementLib/Three-Phase V-I Measurement  VoltageMeasurement=phase-to-ground  SetLabelV=off  LabelV=Vabc  Vpu=off  VpuLL=off  CurrentMeasurement=no  SetLabelI=off  LabelI=Iabc  Ipu=off  Pbase=100e6  Vbase=500e3  OutputType=Complex  PhasorSimulation=off  PSBequivalent=0
  Universal Bridge : spsUniversalBridgeLib/Universal Bridge  Arms=3  SnubberResistance=1e5  SnubberCapacitance=inf  Device=Average-model based VSC  Ron=1e-3  Lon=0  ForwardVoltages="[  0  0  ]"  ForwardVoltage=0  GTOparameters=[ 10e-6 , 20e-6 ]  IGBTparameters=[ 1e-6 , 2e-6 ]  Measurements=None  Measurements_2=None  converterType=Rectifier
  Voltage Measurement : spsVoltageMeasurementLib/Voltage Measurement  PhasorSimulation=off  OutputType=Complex  PSBequivalent=0
  a : PMIOPort  Side=Right
  b : PMIOPort  Port=2  Side=Right
  c : PMIOPort  Port=3  Side=Right
  v_cabc : Outport
  i_tabc : Outport  Port=2
  v_tabc : Outport  Port=3
  v_dc : Outport  Port=4
  wires:
  Three-Phase V-I Measurement/2 -> i_tabc/1
  Three-Phase V-I Measurement2/1 -> v_cabc/1
  Three-Phase V-I Measurement/1 -> v_tabc/1
  eta_abc/1 -> Universal Bridge/1
  Voltage Measurement/1 -> v_dc/1
  connections:
  Three-Phase V-I Measurement/RConn3 -- Three-Phase Series RLC Branch/LConn3
  Three-Phase V-I Measurement/LConn2 -- Universal Bridge/LConn2
  Three-Phase V-I Measurement/RConn1 -- Three-Phase Series RLC Branch/LConn1
  Three-Phase V-I Measurement2/LConn3 -- Three-Phase Series RLC Branch/RConn3 -- Three-Phase Series RLC Branch1/LConn3
  DC Voltage Source/RConn1 -- Voltage Measurement/LConn1 -- Universal Bridge/RConn1
  DC Voltage Source/LConn1 -- Voltage Measurement/LConn2 -- Universal Bridge/RConn2
  Three-Phase Series RLC Branch2/LConn2 -- Three-Phase V-I Measurement2/RConn2
  Three-Phase Series RLC Branch2/LConn1 -- Three-Phase V-I Measurement2/RConn3
  Three-Phase Series RLC Branch1/LConn2 -- Three-Phase V-I Measurement2/LConn2 -- Three-Phase Series RLC Branch/RConn2
  Three-Phase Series RLC Branch/LConn2 -- Three-Phase V-I Measurement/RConn2
  Three-Phase V-I Measurement/LConn1 -- Universal Bridge/LConn1
  Three-Phase Series RLC Branch1/LConn1 -- Three-Phase V-I Measurement2/LConn1 -- Three-Phase Series RLC Branch/RConn1
  Three-Phase V-I Measurement2/RConn1 -- Three-Phase Series RLC Branch2/LConn3
  Three-Phase Series RLC Branch2/RConn1 -- Three-Phase Series RLC Branch2/RConn3 -- Three-Phase Series RLC Branch2/RConn2
  Three-Phase V-I Measurement/LConn3 -- Universal Bridge/LConn3
  a/RConn1 -- Three-Phase Series RLC Branch1/RConn1
  b/RConn1 -- Three-Phase Series RLC Branch1/RConn2
  Three-Phase Series RLC Branch1/RConn3 -- c/RConn1

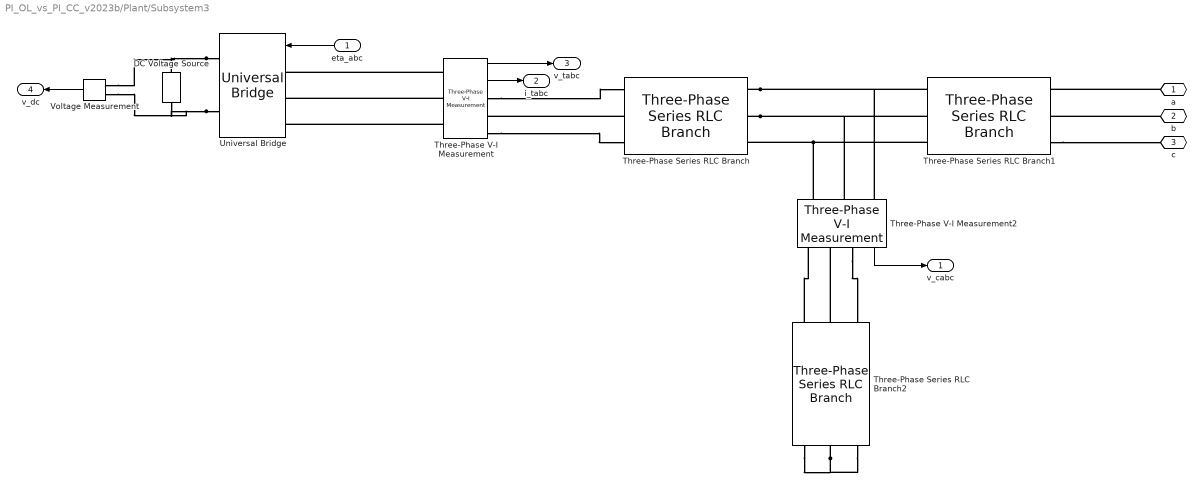
== system PI_OL_vs_PI_CC_v2023b/Plant/Subsystem3 ==
  eta_abc : Inport
  DC Voltage Source : spsDCVoltageSourceLib/DC Voltage Source  Amplitude=v_dc  Measurements=None
  Three-Phase Series RLC Branch : spsThreePhaseSeriesRLCBranchLib/Three-Phase Series RLC Branch  LConnTagsString=A|B|C  RConnTagsString=A|B|C  BranchType=RL  Resistance=R_t2  Inductance=L_t2  Capacitance=1e-6  Measurements=None
  Three-Phase Series RLC Branch1 : spsThreePhaseSeriesRLCBranchLib/Three-Phase Series RLC Branch  LConnTagsString=A|B|C  RConnTagsString=A|B|C  BranchType=RL  Resistance=R_s2  Inductance=L_s2  Capacitance=1e-6  Measurements=None
  Three-Phase Series RLC Branch2 : spsThreePhaseSeriesRLCBranchLib/Three-Phase Series RLC Branch  LConnTagsString=A|B|C  RConnTagsString=A|B|C  BranchType=RC  Resistance=R_d2  Inductance=L_t  Capacitance=C_2  Measurements=None
  Three-Phase V-I Measurement : spsThreePhaseVIMeasurementLib/Three-Phase V-I Measurement  VoltageMeasurement=phase-to-ground  SetLabelV=off  LabelV=Vabc  Vpu=off  VpuLL=off  CurrentMeasurement=yes  SetLabelI=off  LabelI=Iabc  Ipu=off  Pbase=100e6  Vbase=500e3  OutputType=Complex  PhasorSimulation=off  PSBequivalent=0
  Three-Phase V-I Measurement2 : spsThreePhaseVIMeasurementLib/Three-Phase V-I Measurement  VoltageMeasurement=phase-to-ground  SetLabelV=off  LabelV=Vabc  Vpu=off  VpuLL=off  CurrentMeasurement=no  SetLabelI=off  LabelI=Iabc  Ipu=off  Pbase=100e6  Vbase=500e3  OutputType=Complex  PhasorSimulation=off  PSBequivalent=0
  Universal Bridge : spsUniversalBridgeLib/Universal Bridge  Arms=3  SnubberResistance=1e5  SnubberCapacitance=inf  Device=Average-model based VSC  Ron=1e-3  Lon=0  ForwardVoltages="[  0  0  ]"  ForwardVoltage=0  GTOparameters=[ 10e-6 , 20e-6 ]  IGBTparameters=[ 1e-6 , 2e-6 ]  Measurements=None  Measurements_2=None  converterType=Rectifier
  Voltage Measurement : spsVoltageMeasurementLib/Voltage Measurement  PhasorSimulation=off  OutputType=Complex  PSBequivalent=0
  a : PMIOPort  Side=Right
  b : PMIOPort  Port=2  Side=Right
  c : PMIOPort  Port=3  Side=Right
  v_cabc : Outport
  i_tabc : Outport  Port=2
  v_tabc : Outport  Port=3
  v_dc : Outport  Port=4
  wires:
  Voltage Measurement/1 -> v_dc/1
  eta_abc/1 -> Universal Bridge/1
  Three-Phase V-I Measurement/1 -> v_tabc/1
  Three-Phase V-I Measurement2/1 -> v_cabc/1
  Three-Phase V-I Measurement/2 -> i_tabc/1
  connections:
  Three-Phase Series RLC Branch1/RConn3 -- c/RConn1
  b/RConn1 -- Three-Phase Series RLC Branch1/RConn2
  a/RConn1 -- Three-Phase Series RLC Branch1/RConn1
  Three-Phase V-I Measurement/LConn3 -- Universal Bridge/LConn3
  Three-Phase Series RLC Branch2/RConn2 -- Three-Phase Series RLC Branch2/RConn3 -- Three-Phase Series RLC Branch2/RConn1
  Three-Phase V-I Measurement2/RConn1 -- Three-Phase Series RLC Branch2/LConn3
  Three-Phase Series RLC Branch/RConn1 -- Three-Phase V-I Measurement2/LConn1 -- Three-Phase Series RLC Branch1/LConn1
  Three-Phase V-I Measurement/LConn1 -- Universal Bridge/LConn1
  Three-Phase Series RLC Branch/LConn2 -- Three-Phase V-I Measurement/RConn2
  Three-Phase Series RLC Branch/RConn2 -- Three-Phase V-I Measurement2/LConn2 -- Three-Phase Series RLC Branch1/LConn2
  Three-Phase Series RLC Branch2/LConn1 -- Three-Phase V-I Measurement2/RConn3
  Three-Phase Series RLC Branch2/LConn2 -- Three-Phase V-I Measurement2/RConn2
  Universal Bridge/RConn2 -- Voltage Measurement/LConn2 -- DC Voltage Source/LConn1
  Universal Bridge/RConn1 -- Voltage Measurement/LConn1 -- DC Voltage Source/RConn1
  Three-Phase Series RLC Branch1/LConn3 -- Three-Phase Series RLC Branch/RConn3 -- Three-Phase V-I Measurement2/LConn3
  Three-Phase V-I Measurement/RConn1 -- Three-Phase Series RLC Branch/LConn1
  Three-Phase V-I Measurement/LConn2 -- Universal Bridge/LConn2
  Three-Phase V-I Measurement/RConn3 -- Three-Phase Series RLC Branch/LConn3

== matlab function PI_OL_vs_PI_CC_v2023b/Control PI_VC/MATLAB Function2 ==
  data: theta input size=1; dq output; abc input
function dq  = fcn(theta,abc)
%#codegen

T_p = 2.0/3.0*[[ cos(theta), cos(theta-2.0/3.0*pi), cos(theta+2.0/3.0*pi)];
               [-sin(theta),-sin(theta-2.0/3.0*pi),-sin(theta+2.0/3.0*pi)]];
           
dq=T_p*abc;

== matlab function PI_OL_vs_PI_CC_v2023b/Control PI_CC/MATLAB Function4 ==
  data: theta input size=1; dq output; abc input
function dq  = fcn(theta,abc)
%#codegen

T_p = 2.0/3.0*[[ cos(theta), cos(theta-2.0/3.0*pi), cos(theta+2.0/3.0*pi)];
               [-sin(theta),-sin(theta-2.0/3.0*pi),-sin(theta+2.0/3.0*pi)]];
           
dq=T_p*abc;

== matlab function PI_OL_vs_PI_CC_v2023b/Control PI_CC/MATLAB Function5 ==
  data: theta input size=1; abc output size=3; dq input
function abc  = fcn(theta,dq)
%#codegen

T_p_inv = [[            cos(theta),            -sin(theta)];
           [ cos(theta-2.0/3.0*pi), -sin(theta-2.0/3.0*pi)];
           [ cos(theta+2.0/3.0*pi), -sin(theta+2.0/3.0*pi)]];
           
abc=T_p_inv*dq;

== matlab function PI_OL_vs_PI_CC_v2023b/Control PI_CC/PLL/MATLAB Function1 ==
  data: theta input size=1; dq output; abc input
function dq  = fcn(theta,abc)
%#codegen

T_p = 2.0/3.0*[[ cos(theta), cos(theta-2.0/3.0*pi), cos(theta+2.0/3.0*pi)];
               [-sin(theta),-sin(theta-2.0/3.0*pi),-sin(theta+2.0/3.0*pi)]];
           
dq=T_p*abc;

== matlab function PI_OL_vs_PI_CC_v2023b/Control PI_CC/VSG ==
  data: p_m_ref input; q_s_ref input; i_sdq input; i_sdq_ref output size=2; omega_rads output; v_sdq input; params input; omega_base input; x input; dx output
function [i_sdq_ref,omega_rads,dx] = ctrl_3(p_m_ref,q_s_ref,i_sdq,v_sdq,params,omega_base,x)
%Initialization
i_sdq_ref = [0;0];
fault_flag = 0;
e_0 = 1.0;

% parameters
S_b = params(1);
U_b = params(2);
K_p = params(3);
T_p = params(4);
K_q = params(5);
T_q = params(6);
X = params(7);
R = params(8);

%Base value
I_b = S_b/(sqrt(3)*U_b);
I_bdq = I_b*sqrt(2); 
U_bdq = U_b*(sqrt(2/3));

%Current and voltage in pu
i_sd = i_sdq(1)/I_bdq; % input in SI that is coverted to pu
i_sq = i_sdq(2)/I_bdq; % input in SI that is coverted to pu
v_sd = v_sdq(1)/U_bdq; % input in SI that is coverted to pu
v_sq = v_sdq(2)/U_bdq; % input in SI that is coverted to pu

%Active power en pu
p_s = i_sd*v_sd + i_sq*v_sq; % pu
q_s = i_sd*v_sq - i_sq*v_sd; % pu 

% from the integrator to the states
phi  = x(1);
xi_p = x(2);
xi_q = x(3);
omega_fil = x(4);

%error of active and reactive power
epsilon_p = (p_m_ref - p_s)*(1.0-fault_flag);
epsilon_q = q_s_ref - q_s;

%omega VSG
omega = K_p*(epsilon_p + xi_p/T_p) + omega_base; 
omega_rads = 2.0*pi*50.0*omega;
%Derivative outputs
dphi =  omega_rads;
dxi_p = epsilon_p;
dxi_q = epsilon_q; 
domega_rads = 1.0/1.0*(2.0*pi*50.0*omega - omega_fil);

%Voltage increase
DV =   K_q*(epsilon_q + xi_q/T_q); 

%Saturation of DV
DV_sat = DV;
if DV_sat > 0.1 
    DV_sat = 0.1;
    dxi_q = 0.0;
end
if DV_sat < -0.1 
    DV_sat = -0.1;
    dxi_q = 0.0;
end   

%Electromotive force of VSG
e = e_0 + DV_sat; 

%Virtual impdance
i_sd = -(X*e + R*v_sd + X*v_sq)/(R^2 + X^2);
i_sq = -(R*e + R*v_sq - X*v_sd)/(R^2 + X^2);

%Current references in A
i_sdq_ref(1) = i_sd*I_bdq;
i_sdq_ref(2) = i_sq*I_bdq;


% from derivatives to the integrator
dx = [dphi;dxi_p;dxi_q;domega_rads];

== matlab function PI_OL_vs_PI_CC_v2023b/Control PI_CC/MATLAB Function ==
  data: i_s_abc input; i_s_abc_ref output; time input
function i_s_abc_ref = fcn(i_s_abc,time)
i_s_abc_ref = [0;0];

if time >1
    i_s_abc_ref = [i_s_abc(1);i_s_abc(2)];
end

== matlab function PI_OL_vs_PI_CC_v2023b/Control PI_VC/PLL/MATLAB Function1 ==
  data: theta input size=1; dq output; abc input
function dq  = fcn(theta,abc)
%#codegen

T_p = 2.0/3.0*[[ cos(theta), cos(theta-2.0/3.0*pi), cos(theta+2.0/3.0*pi)];
               [-sin(theta),-sin(theta-2.0/3.0*pi),-sin(theta+2.0/3.0*pi)]];
           
dq=T_p*abc;

== matlab function PI_OL_vs_PI_CC_v2023b/Control PI_VC/VSG ==
  data: e_0 input; p_m_ref input; q_s_ref input; i_sdq input; v_sdq input; v_mdq_ref output size=2; omega_rads output; params input; omega_base input; x input; dx output
function [v_mdq_ref,omega_rads,dx] = ctrl_3(e_0,p_m_ref,q_s_ref,i_sdq,v_sdq,params,omega_base,x)
%Initialization
v_mdq_ref = [0;0];
fault_flag = 0;

% parameters
S_b = params(1);
U_b = params(2);
K_p = params(3);
T_p = params(4);
K_q = params(5);
T_q = params(6);
X = params(7);
R = params(8);

%Base value
I_b = S_b/(sqrt(3)*U_b);
I_bdq = I_b*sqrt(2); 
U_bdq = U_b*(sqrt(2/3));

%Current and voltage in pu

v_sd = v_sdq(1)/U_bdq; % input in SI that is coverted to pu
v_sq = v_sdq(2)/U_bdq; % input in SI that is coverted to pu
i_sd = i_sdq(1)/I_bdq; % input in SI that is coverted to pu
i_sq = i_sdq(2)/I_bdq; % input in SI that is coverted to pu
%Active power en pu
p_s = i_sd*v_sd + i_sq*v_sq; % pu
q_s = i_sd*v_sq - i_sq*v_sd; % pu 

% from the integrator to the states
phi  = x(1);
xi_p = x(2);
xi_q = x(3);
omega_fil = x(4);

%error of active and reactive power
epsilon_p = (p_m_ref - p_s)*(1.0-fault_flag);
epsilon_q = q_s_ref - q_s;

%omega VSG
omega = K_p*(epsilon_p + xi_p/T_p) + omega_base; 
omega_rads = 2.0*pi*50.0*omega;
%Derivative outputs
dphi =  omega_rads;
dxi_p = epsilon_p;
dxi_q = epsilon_q; 
domega_rads = 1.0/1.0*(2.0*pi*50.0*omega - omega_fil);

%Voltage increase
DV =   K_q*(epsilon_q + xi_q/T_q*1); 

%Saturation of DV
DV_sat = DV;
if DV_sat > 0.1 
    DV_sat = 0.1;
    dxi_q = 0.0;
end
if DV_sat < -0.1 
    DV_sat = -0.1;
    dxi_q = 0.0;
end   

%Electromotive force of VSG
e = e_0 + DV_sat; 
e_d =0;
e_q = -e;
%Virtual impdance
v_md = e_d ;
v_mq = e_q ;

%Current references in A
v_mdq_ref(1) = v_md*U_bdq;
v_mdq_ref(2) = v_mq*U_bdq;


% from derivatives to the integrator
dx = [dphi;dxi_p;dxi_q;domega_rads];

== matlab function PI_OL_vs_PI_CC_v2023b/Control PI_VC/MATLAB Function3 ==
  data: theta input size=1; dq output; abc input
function dq  = fcn(theta,abc)
%#codegen

T_p = 2.0/3.0*[[ cos(theta), cos(theta-2.0/3.0*pi), cos(theta+2.0/3.0*pi)];
               [-sin(theta),-sin(theta-2.0/3.0*pi),-sin(theta+2.0/3.0*pi)]];
           
dq=T_p*abc;

== matlab function PI_OL_vs_PI_CC_v2023b/Control PI_VC/MATLAB Function4 ==
  data: theta input size=1; dq output; abc input
function dq  = fcn(theta,abc)
%#codegen

T_p = 2.0/3.0*[[ cos(theta), cos(theta-2.0/3.0*pi), cos(theta+2.0/3.0*pi)];
               [-sin(theta),-sin(theta-2.0/3.0*pi),-sin(theta+2.0/3.0*pi)]];
           
dq=T_p*abc;

== matlab function PI_OL_vs_PI_CC_v2023b/Control PI_VC/MATLAB Function5 ==
  data: theta input size=1; abc output size=3; dq input
function abc  = fcn(theta,dq)
%#codegen

T_p_inv = [[            cos(theta),            -sin(theta)];
           [ cos(theta-2.0/3.0*pi), -sin(theta-2.0/3.0*pi)];
           [ cos(theta+2.0/3.0*pi), -sin(theta+2.0/3.0*pi)]];
           
abc=T_p_inv*dq;

== matlab function PI_OL_vs_PI_CC_v2023b/Control PI_CC/Current Control ==
  data: i_sdq_ref input; i_sdq input; eta_dq output size=2; v_sdq input; v_dc input; omega input; params input; x input; dx output
function [eta_dq,dx] = ctrl_vsc(i_sdq_ref,i_sdq,v_sdq,v_dc,omega,params,x)

% parameters
L_t = params(2);
L_s = params(4);
K_p = params(5);
K_i = params(6);

%References
i_sd_ref = i_sdq_ref(1);
i_sq_ref = i_sdq_ref(2);

i_sd = i_sdq(1);
i_sq = i_sdq(2);
v_sd = v_sdq(1);
v_sq = v_sdq(2);

% from the integrator to the states
xi_isd = x(1);
xi_isq = x(2);


% auxiliar
e_isd = i_sd_ref - i_sd;
e_isq = i_sq_ref - i_sq;

% derivatives
dxi_isd = e_isd;
dxi_isq = e_isq;


% auxiliar
u_d = K_p*e_isd + K_i*xi_isd;
u_q = K_p*e_isq + K_i*xi_isq;
L = L_t + L_s ;

% outputs
eta_d = 2/v_dc*(u_d +  - L*omega*i_sq + v_sd);
eta_q = 2/v_dc*(u_q +  + L*omega*i_sd + v_sq);
eta_dq = [eta_d ; eta_q];


% from derivatives to the integrator
dx = [dxi_isd;dxi_isq];

== matlab function PI_OL_vs_PI_CC_v2023b/Control PI_CC/MATLAB Function3 ==
  data: theta input size=1; dq output; abc input
function dq  = fcn(theta,abc)
%#codegen

T_p = 2.0/3.0*[[ cos(theta), cos(theta-2.0/3.0*pi), cos(theta+2.0/3.0*pi)];
               [-sin(theta),-sin(theta-2.0/3.0*pi),-sin(theta+2.0/3.0*pi)]];
           
dq=T_p*abc;

== matlab function PI_OL_vs_PI_CC_v2023b/Control PI_VC/MATLAB Function1 ==
  data: theta input size=1; dq output; abc input
function dq  = fcn(theta,abc)
%#codegen

T_p = 2.0/3.0*[[ cos(theta), cos(theta-2.0/3.0*pi), cos(theta+2.0/3.0*pi)];
               [-sin(theta),-sin(theta-2.0/3.0*pi),-sin(theta+2.0/3.0*pi)]];
           
dq=T_p*abc;
